simulink model "PID_Controller_2"  (R2018b)
settings: Solver=FixedStepAuto  StartTime=0.0  StopTime=10.0  FixedStep=0.01  RelTol=1e-3
settings Model: Creator=mokeam  LastModifiedBy=mokeam

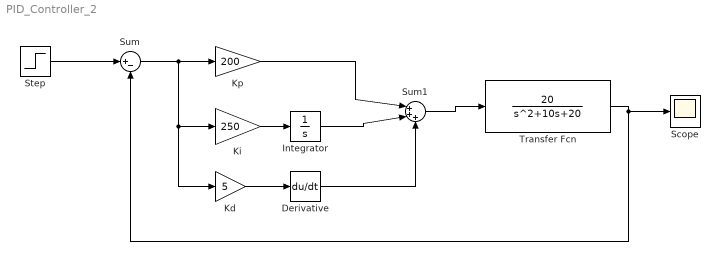
== system PID_Controller_2 ==
  Derivative : Derivative
  Integrator : Integrator
  Kd : Gain  Gain=5
  Ki : Gain  Gain=250
  Kp : Gain  Gain=200
  Scope : Scope
  Step : Step  Time=0  SampleTime=0
  Sum : Sum  Inputs=|+-
  Sum1 : Sum  Inputs=|+++
  Transfer Fcn : TransferFcn  Numerator=[20]  Denominator=[1 10 20]
  wires:
  Step/1 -> Sum/1
  Sum/1 -> Kd/1, Ki/1, Kp/1
  Kd/1 -> Derivative/1
  Ki/1 -> Integrator/1
  Kp/1 -> Sum1/1
  Integrator/1 -> Sum1/2
  Derivative/1 -> Sum1/3
  Sum1/1 -> Transfer Fcn/1
  Transfer Fcn/1 -> Scope/1, Sum/2
